simulink model "atti"  (R2022b)
settings: Solver=FixedStepAuto  StartTime=0.0  StopTime=T  RelTol=1e-3
values from neighbouring files (symbols this model uses):
  dt = 1/fs    (= 0.005)    [attitude_main.m]
  dwd = [dwd1', dwd2', dwd3']    [attitude_main.m]    (also in desired_trajectory.mat = [1 1 1 1 1 1 1 1 1 1 1 1 ... (6003 elements, 2001x3)]; main.m = [dwd1', 0*t', 0*t'])
  J = diag([0.029 0.029 0.055])    [attitude_main.m]
  K = place(A, B, desired_poles)    [attitude_main.m]
  Rd = R_sequence    [attitude_main.m]    (also in desired_trajectory.mat = [1 0 0 0 1 0 0 0 1 1 0 0 ... (18009 elements, 3x3x2001)]; main.m = eul2rotm([ 0*t', 0*t',Rd1']))
  wd = [wd1', wd2', wd3']    [attitude_main.m]    (also in desired_trajectory.mat = [0 0.005 0.01 0.015 0.02 0.025 0.03 0.035 0.04 0.045 0.05 0.; main.m = [wd1', 0*t', 0*t'])
libraries: simulink x6, shared6dof x1, aerolibutil x1
settings Model: Creator=zzy  LastModifiedBy=MoC
settings DataIOCC: ReturnWorkspaceOutputs=off

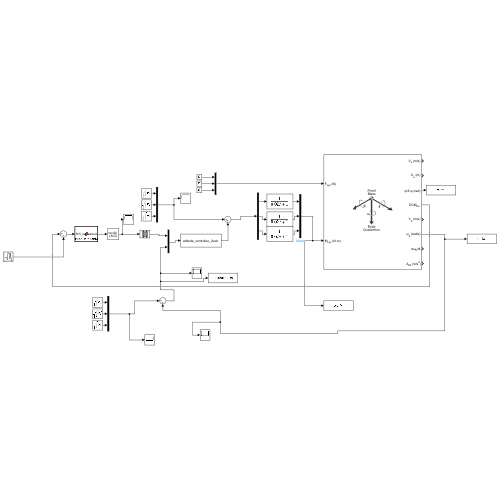
[thumbnail: Simulink's stored preview of the top-level diagram]
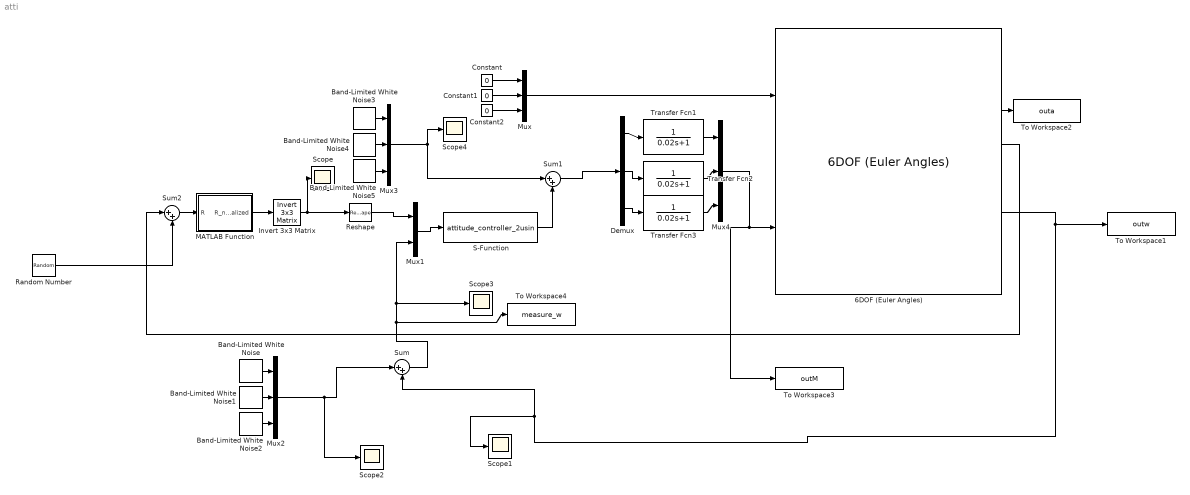
== system atti ==
  6DOF (Euler Angles) : shared6dof/6DOF (Euler Angles)  units=Metric (MKS)  mtype=Fixed  rep=Quaternion  xme_0=[0 0 0]  Vm_0=[0 0 0]  eul_0=[0 0 0]  pm_0=[0 0 0]  mass_0=1  mass_e=0.5  mass_f=2.0  inertia=J  inertia_e=eye(3)  inertia_f=2*eye(3)  k_quat=1.0  vre_flag=on  abi_flag=off  aMode=0  xme_statename=''  Vm_statename=''  eul_statename=''  quat_statename=''  pm_statename=''  mass_statename=''
  Band-Limited White Noise : simulink/Sources/Band-Limited White Noise  Cov=0.00004  Ts=dt  seed=[2341]  VectorParams1D=off
  Band-Limited White Noise1 : simulink/Sources/Band-Limited White Noise  Cov=0.00004  Ts=dt  seed=[23341]  VectorParams1D=off
  Band-Limited White Noise2 : simulink/Sources/Band-Limited White Noise  Cov=0.00004  Ts=dt  seed=[20341]  VectorParams1D=off
  Band-Limited White Noise3 : simulink/Sources/Band-Limited White Noise  Cov=0.00001  Ts=dt  seed=35234  VectorParams1D=off
  Band-Limited White Noise4 : simulink/Sources/Band-Limited White Noise  Cov=0.00004  Ts=dt  seed=245645  VectorParams1D=off
  Band-Limited White Noise5 : simulink/Sources/Band-Limited White Noise  Cov=0.000004  Ts=dt  seed=456445  VectorParams1D=off
  Constant : Constant  Value=0
  Constant1 : Constant  Value=0
  Constant2 : Constant  Value=0
  Demux : Demux  Outputs=3
  Invert 3x3 Matrix : aerolibutil/Invert  3x3 Matrix
  MATLAB Function : MATLAB Function  TreatAsAtomicUnit=on
  Mux{,2..4} (4 alike) : Mux  Inputs=3
  Mux1 : Mux  Inputs=2
  Random Number : RandomNumber  Variance=0.01  SampleTime=dt
  Reshape : Reshape  OutputDimensionality=Column vector (2-D)
  S-Function : S-Function  FunctionName=attitude_controller_2usin  Parameters=dt,Rd,wd,dwd,J,K  SFunctionDeploymentMode=off  EnableBusSupport=off
  Scope{,1..4} (5 alike) : Scope
  Sum : Sum  Inputs=|++
  Sum1 : Sum  Inputs=|++
  Sum2 : Sum  Inputs=|++
  To Workspace1 : ToWorkspace  VariableName=outw  SampleTime=-1
      settings: Save2DSignal=2-D array (concatenate along first dimension)
  To Workspace2 : ToWorkspace  VariableName=outa  SampleTime=-1
      settings: Save2DSignal=2-D array (concatenate along first dimension)
  To Workspace3 : ToWorkspace  VariableName=outM  SampleTime=-1
      settings: Save2DSignal=2-D array (concatenate along first dimension)
  To Workspace4 : ToWorkspace  VariableName=measure_w  SampleTime=-1
      settings: Save2DSignal=2-D array (concatenate along first dimension)
  Transfer Fcn1 : TransferFcn  Denominator=[0.02 1]
  Transfer Fcn2 : TransferFcn  Denominator=[0.02 1]
  Transfer Fcn3 : TransferFcn  Denominator=[0.02 1]
  wires:
  Constant1/1 -> Mux/2
  Constant/1 -> Mux/1
  Constant2/1 -> Mux/3
  Mux/1 -> 6DOF (Euler Angles)/1
  S-Function/1 -> Sum1/2
  6DOF (Euler Angles)/6 -> Sum/2, Scope1/1, To Workspace1/1
  Invert 3x3 Matrix/1 -> Scope/1, Reshape/1
  Mux1/1 -> S-Function/1
  Reshape/1 -> Mux1/1
  6DOF (Euler Angles)/3 -> To Workspace2/1
  Sum/1 -> Mux1/2, Scope3/1, To Workspace4/1
  Band-Limited White Noise/1 -> Mux2/1
  Band-Limited White Noise1/1 -> Mux2/2
  Band-Limited White Noise2/1 -> Mux2/3
  Mux2/1 -> Scope2/1, Sum/1
  Band-Limited White Noise4/1 -> Mux3/2
  Band-Limited White Noise5/1 -> Mux3/3
  Band-Limited White Noise3/1 -> Mux3/1
  Mux3/1 -> Scope4/1, Sum1/1
  Sum1/1 -> Demux/1
  Mux4/1 -> To Workspace3/1, 6DOF (Euler Angles)/2
  Transfer Fcn2/1 -> Mux4/2
  Transfer Fcn1/1 -> Mux4/1
  Transfer Fcn3/1 -> Mux4/3
  Demux/3 -> Transfer Fcn3/1
  Demux/2 -> Transfer Fcn2/1
  Demux/1 -> Transfer Fcn1/1
  Random Number/1 -> Sum2/2
  6DOF (Euler Angles)/4 -> Sum2/1
  Sum2/1 -> MATLAB Function/1(R)
  MATLAB Function/1(R_normalized) -> Invert 3x3 Matrix/1

== matlab function atti/MATLAB Function ==
  data: R input; R_normalized output
function R_normalized = normalizeRotationMatrix(R)
% Normalize a rotation matrix using SVD
    [U, ~, V] = svd(R);
    R_normalized = U * V';
end
